simulink model "F2"  (Simulink 7.4)
settings: Solver=ode45  StartTime=0.0  StopTime=10.0  RelTol=1e-3
settings Model: Creator=alex  LastModifiedBy=alesch
settings OptimizationCC: InlineParams=on

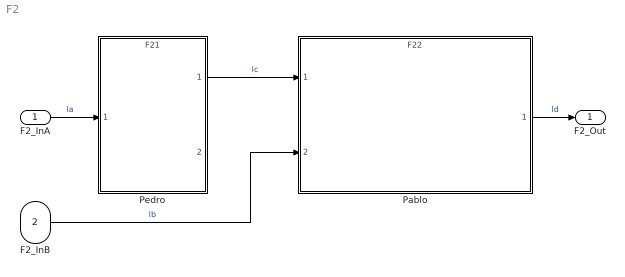
== system F2 ==
  F2_InA : Inport
  F2_InB : Inport  Port=2  OutDataType=fixdt(1, 16)  OutScaling=2^0
  Pablo : ModelReference  ModelNameDialog=F22  SimulationMode=Accelerator  ModelReferenceVersion=1.2  CopyOfModelName=F22
  Pedro : ModelReference  ModelNameDialog=F21  SimulationMode=Accelerator  ModelReferenceVersion=1.4  CopyOfModelName=F21
  F2_Out : Outport
  wires:
  F2_InA/1 -> Pedro/1  "la"
  Pedro/1 -> Pablo/1  "lc"
  Pablo/1 -> F2_Out/1  "ld"
  F2_InB/1 -> Pablo/2  "lb"
